simulink subsystem "dipole_magnetic_model"  (R2023b)
settings: Solver=VariableStepAuto  StartTime=0.0  StopTime=10.0  RelTol=1e-3
settings Model: Creator=pierb  LastModifiedBy=pierb

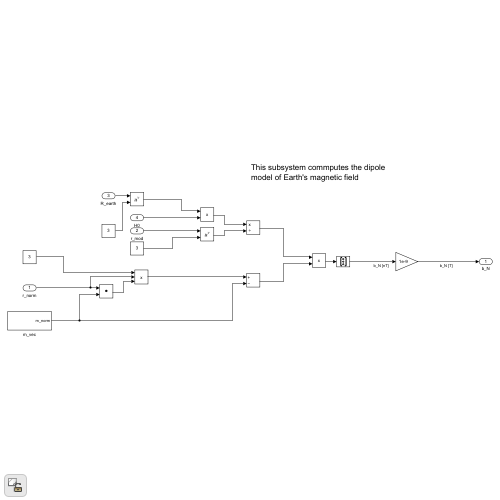
[thumbnail: Simulink's stored preview of the top-level diagram]
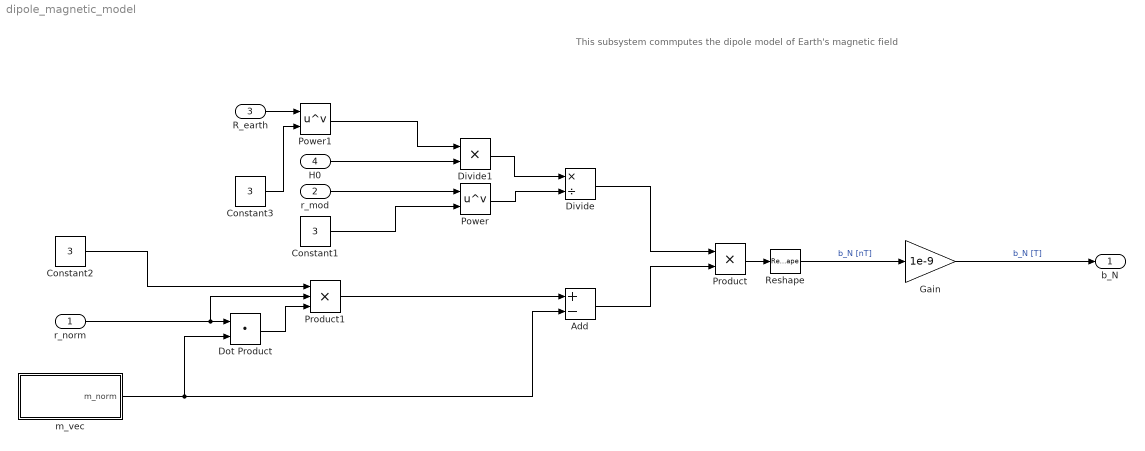
== system dipole_magnetic_model ==
  note: This subsystem commputes the dipole
      | model of Earth's magnetic field
  r_norm : Inport
  r_mod : Inport  Port=2
  R_earth : Inport  Port=3
  H0 : Inport  Port=4
  Add : Sum  Inputs=+-
  Constant1 : Constant  Value=3
  Constant2 : Constant  Value=3
  Constant3 : Constant  Value=3
  Divide : Product  Inputs=*/
  Divide1 : Product  Inputs=**
  Dot Product : DotProduct  OutDataTypeStr=Inherit: Inherit via internal rule
  Gain : Gain  Gain=1e-9
  Power : Math  Operator=pow
  Power1 : Math  Operator=pow
  Product : Product
  Product1 : Product  Inputs=3
  Reshape : Reshape  OutputDimensionality=Column vector (2-D)
  m_vec : Subsystem
  b_N : Outport
  wires:
  m_vec/1(m_norm) -> Add/2, Dot Product/2
  Reshape/1 -> Gain/1  "b_N [nT]"
  Constant2/1 -> Product1/1
  Product1/1 -> Add/1
  r_mod/1 -> Power/1
  Dot Product/1 -> Product1/3
  Add/1 -> Product/2
  Constant1/1 -> Power/2
  Divide/1 -> Product/1
  Power/1 -> Divide/2
  r_norm/1 -> Dot Product/1, Product1/2
  Product/1 -> Reshape/1
  Gain/1 -> b_N/1  "b_N [T]"
  R_earth/1 -> Power1/1
  Constant3/1 -> Power1/2
  H0/1 -> Divide1/2
  Power1/1 -> Divide1/1
  Divide1/1 -> Divide/1

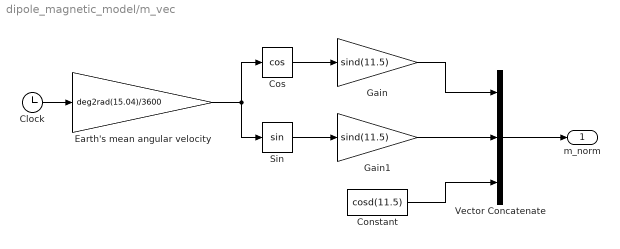
== system dipole_magnetic_model/m_vec ==
  Clock : Clock
  Constant : Constant  Value=cosd(11.5)
  Cos : Trigonometry  Operator=cos
  Earth's mean angular velocity : Gain  Gain=deg2rad(15.04)/3600
  Gain : Gain  Gain=sind(11.5)
  Gain1 : Gain  Gain=sind(11.5)
  Sin : Trigonometry
  Vector Concatenate : Concatenate  NumInputs=3
  m_norm : Outport
  wires:
  Gain/1 -> Vector Concatenate/1
  Gain1/1 -> Vector Concatenate/2
  Sin/1 -> Gain1/1
  Cos/1 -> Gain/1
  Earth's mean angular velocity/1 -> Sin/1, Cos/1
  Clock/1 -> Earth's mean angular velocity/1
  Constant/1 -> Vector Concatenate/3
  Vector Concatenate/1 -> m_norm/1
